simulink model "EPT"  (R2019b)
settings: Solver=FixedStepDiscrete  StartTime=0.0  StopTime=5  FixedStep=0.005  RelTol=1e-3  EnableMultiTasking=on
PreLoadFcn:
  | try, model_open; catch, disp('Error occurred while executing model pre-load callback: model_open.m'); disp('Please assure that the MATLAB working directory is set to the model directory before opening.'); end
InitFcn:
  | try, model_open; catch, end
undefined symbols (not defined in the file or in its folder): Bridge, GCM, H, ln, raptor_get_param_eval, raptor_get_safe_string, raptor_xcp_function
libraries: Raptor_lib x2810, simulink x374, hdlsllib x19
(part 13 of 45)

== system EPT/Foreground_TimeBase_5ms/CAN/CAN1_exec/BCU vs RMDA-BMS/Remote DAG2-5E6 ==
  Trigger : TriggerPort  VariantControl=Variant  PortDimensions=1
  Bitwise Operator : simulink/Logic and Bit Operations/Bitwise Operator  logicop=AND  UseBitMask=on  BitMask=hex2dec('f0')  BitMaskRealWorld=Stored Integer
  Bitwise Operator1 : simulink/Logic and Bit Operations/Bitwise Operator  logicop=AND  UseBitMask=on  BitMask=hex2dec('0f')  BitMaskRealWorld=Stored Integer
  Data Type Conversion{,1..5} (6 alike) : DataTypeConversion
  Fcn1 : Fcn  Expr=(u(1)+12.5)/0.5
  Shift Arithmetic1 : ArithShift  BitShiftNumber=4  BitShiftDirection=Right
  raptor_can_txmsg : Raptor_lib/CAN/raptor_can_txmsg  canDefinition=struct('dbcFile', 'BCUvsRMDA_CMU.dbc','message', 'RemoteDAG_5E6','comment', '','signals', {{'CMU2_EW_Level3_Hbyte','CMU2_EW_Level3_Lbyte','CMU2_FCC','CMU2_Mode','CMU2_RSOC','CMU2_Rcap'}},'enabled', [ 1 1 1 1 1 1;],'canBus', '''CAN1''','messageID', [ 1510;],'idMask', [ 536870911;],'payloadMask', [],'payloadValue', [],'period', [ 0;],'mailbox', '','queueSize', [ 1;],'label', [ 0;],'ver', [ 2;],'showID', [ 0;],'showRaw', [ 0;],'fill', [ 0;],'editID', [ 0;],'signalOrder', [ 1;])  canBus='CAN1'  queueSize=1  payloadMask=[]  payloadValue=[]  period=0  showID=0  label=0  idMask=hex2dec('1FFFFFFF')  fill=0  id=1510  showRaw=0  signalOrder=1  signalInfo={{struct('Name', 'CMU2_Mode','Startbit', [ 0;],'SignalSize', [ 8;],'ByteOrder', 'BigEndian','ValueType', 'UNSIGNED','Class', 'uint8','Signed', [ 0;],'Factor', [ 1;],'Offset', [ 0;],'Min', [ 0;],'Max', [ 0;],'Units', '','Comment', '','StartBit', [ 0;]),struct('Name', 'CMU2_EW_Level3_Hbyte','Startbit', [ 0;],'SignalSize', [ 8;],'ByteOrder', 'BigEndian','ValueType', 'UNSIGNED','Class', 'uint8','Signed', [ 0;],'Factor', [ 1;],'Offset', [ 0;],'Min', [ 0;],'Max', [ 0;],'Units', '','Comment', '','StartBit', [ 8;]),struct('Name', 'CMU2_EW_Level3_Lbyte','Startbit', [ 0;],'SignalSize', [ 8;],'ByteOrder', 'BigEndian','ValueType', 'UNSIGNED','Class', 'uint8','Signed', [ 0;],'Factor', [ 1;],'Offset', [ 0;],'Min', [ 0;],'Max', [ 0;],'Units', '','Comment', '','StartBit', [ 16;]),struct('Name', 'CMU2_FCC','Startbit', [ 0;],'SignalSize', [ 8;],'ByteOrder', 'BigEndian','ValueType', 'UNSIGNED','Class', 'uint8','Signed', [ 0;],'Factor', [ 1;],'Offset', [ 0;],'Min', [ 0;],'Max', [ 0;],'Units', '','Comment', '','StartBit', [ 32;]),struct('Name', 'CMU2_Rcap','Startbit', [ 0;],'SignalSize', [ 8;],'ByteOrder', 'BigEndian','ValueType', 'UNSIGNED','Class', 'uint8','Signed', [ 0;],'Factor', [ 1;],'Offset', [ 0;],'Min', [ 0;],'Max', [ 0;],'Units', '','Comment', '','StartBit', [ 40;]),struct('Name', 'CMU2_RSOC','Startbit', [ 0;],'SignalSize', [ 8;],'ByteOrder', 'BigEndian','ValueType', 'UNSIGNED','Class', 'uint8','Signed', [ 0;],'Factor', [ 1;],'Offset', [ 0;],'Min', [ 0;],'Max', [ 0;],'Units', '','Comment', '','StartBit', [ 48;])}}
      settings: SourceProductName=Raptor
  raptor_data_read2 : Raptor_lib/Data Storage/raptor_data_read  dataName='Rx_0x200B2A2_FCC'  dataShape=Scalar  idxSource=Input  idxRow=1  idxCol=1
      settings: SourceProductName=Raptor
  raptor_data_read3 : Raptor_lib/Data Storage/raptor_data_read  dataName='Rx_0x200B0A2_CMU2_Status'  dataShape=Scalar  idxSource=Input  idxRow=1  idxCol=1
      settings: SourceProductName=Raptor
  raptor_data_read4 : Raptor_lib/Data Storage/raptor_data_read  dataName='Rx_0x200B2A2_RC'  dataShape=Scalar  idxSource=Input  idxRow=1  idxCol=1
      settings: SourceProductName=Raptor
  raptor_data_read5 : Raptor_lib/Data Storage/raptor_data_read  dataName='Rx_0x200B2A2_RSOC'  dataShape=Scalar  idxSource=Input  idxRow=1  idxCol=1
      settings: SourceProductName=Raptor
  raptor_data_read6 : Raptor_lib/Data Storage/raptor_data_read  dataName='Rx_0x200BAA2_Event3_Error_Code'  dataShape=Scalar  idxSource=Input  idxRow=1  idxCol=1
      settings: SourceProductName=Raptor
  wires:
  Data Type Conversion/1 -> Data Type Conversion2/1
  Shift Arithmetic1/1 -> Data Type Conversion1/1
  raptor_data_read6/1 -> Bitwise Operator/1, Bitwise Operator1/1
  Bitwise Operator1/1 -> Data Type Conversion/1
  raptor_data_read3/1 -> raptor_can_txmsg/4
  Bitwise Operator/1 -> Shift Arithmetic1/1
  raptor_data_read2/1 -> Data Type Conversion5/1
  Data Type Conversion2/1 -> raptor_can_txmsg/2
  Data Type Conversion1/1 -> raptor_can_txmsg/1
  raptor_data_read5/1 -> Fcn1/1
  Data Type Conversion3/1 -> raptor_can_txmsg/6
  raptor_data_read4/1 -> Data Type Conversion3/1
  Data Type Conversion4/1 -> raptor_can_txmsg/5
  Data Type Conversion5/1 -> raptor_can_txmsg/3
  Fcn1/1 -> Data Type Conversion4/1

== system EPT/Foreground_TimeBase_5ms/CAN/CAN1_exec/BCU vs RMDA-BMS/Remote DAG2-5E7 ==
  Trigger : TriggerPort  VariantControl=Variant  PortDimensions=1
  Data Type Conversion{1..4} (4 alike) : DataTypeConversion
  Fcn1 : Fcn  Expr=(u(1)-2)/0.01
  Fcn2 : Fcn  Expr=(u(1)-2)/0.01
  Fcn3 : Fcn  Expr=(u(1)+40)/0.5
  Fcn4 : Fcn  Expr=(u(1)+40)/0.5
  raptor_can_txmsg : Raptor_lib/CAN/raptor_can_txmsg  canDefinition=struct('dbcFile', 'BCUvsRMDA_CMU.dbc','message', 'RemoteDAG_5E7','comment', '','signals', {{'CMU2_Ibp','CMU2_Tcell_Max','CMU2_Tcell_Min','CMU2_Vbp','CMU2_Vcell_Max','CMU2_Vcell_Min'}},'enabled', [ 1 1 1 1 1 1;],'canBus', '''CAN1''','messageID', [ 1511;],'idMask', [ 536870911;],'payloadMask', [],'payloadValue', [],'period', [ 0;],'mailbox', '','queueSize', [ 1;],'label', [ 0;],'ver', [ 2;],'showID', [ 0;],'showRaw', [ 0;],'fill', [ 0;],'editID', [ 0;],'signalOrder', [ 1;])  canBus='CAN1'  queueSize=1  payloadMask=[]  payloadValue=[]  period=0  showID=0  label=0  idMask=hex2dec('1FFFFFFF')  fill=0  id=1511  showRaw=0  signalOrder=1  signalInfo={{struct('Name', 'CMU2_Ibp','Startbit', [ 0;],'SignalSize', [ 16;],'ByteOrder', 'BigEndian','ValueType', 'UNSIGNED','Class', 'uint16','Signed', [ 0;],'Factor', [ 0.02;],'Offset', [ -500;],'Min', [ 0;],'Max', [ 0;],'Units', '','Comment', '','StartBit', [ 8;]),struct('Name', 'CMU2_Vbp','Startbit', [ 0;],'SignalSize', [ 16;],'ByteOrder', 'BigEndian','ValueType', 'UNSIGNED','Class', 'uint16','Signed', [ 0;],'Factor', [ 0.01;],'Offset', [ 0;],'Min', [ 0;],'Max', [ 0;],'Units', '','Comment', '','StartBit', [ 24;]),struct('Name', 'CMU2_Vcell_Max','Startbit', [ 0;],'SignalSize', [ 8;],'ByteOrder', 'BigEndian','ValueType', 'UNSIGNED','Class', 'uint8','Signed', [ 0;],'Factor', [ 1;],'Offset', [ 0;],'Min', [ 0;],'Max', [ 0;],'Units', '','Comment', '','StartBit', [ 32;]),struct('Name', 'CMU2_Vcell_Min','Startbit', [ 0;],'SignalSize', [ 8;],'ByteOrder', 'BigEndian','ValueType', 'UNSIGNED','Class', 'uint8','Signed', [ 0;],'Factor', [ 1;],'Offset', [ 0;],'Min', [ 0;],'Max', [ 0;],'Units', '','Comment', '','StartBit', [ 40;]),struct('Name', 'CMU2_Tcell_Max','Startbit', [ 0;],'SignalSize', [ 8;],'ByteOrder', 'BigEndian','ValueType', 'UNSIGNED','Class', 'uint8','Signed', [ 0;],'Factor', [ 1;],'Offset', [ 0;],'Min', [ 0;],'Max', [ 0;],'Units', '','Comment', '','StartBit', [ 48;]),struct('Name', 'CMU2_Tcell_Min','Startbit', [ 0;],'SignalSize', [ 8;],'ByteOrder', 'BigEndian','ValueType', 'UNSIGNED','Class', 'uint8','Signed', [ 0;],'Factor', [ 1;],'Offset', [ 0;],'Min', [ 0;],'Max', [ 0;],'Units', '','Comment', '','StartBit', [ 56;])}}
      settings: SourceProductName=Raptor
  raptor_data_read : Raptor_lib/Data Storage/raptor_data_read  dataName='Rx_0x200B0A2_Max_Cell_Volt'  dataShape=Scalar  idxSource=Input  idxRow=1  idxCol=1
      settings: SourceProductName=Raptor
  raptor_data_read1 : Raptor_lib/Data Storage/raptor_data_read  dataName='Rx_0x200B0A2_Min_Cell_Volt'  dataShape=Scalar  idxSource=Input  idxRow=1  idxCol=1
      settings: SourceProductName=Raptor
  raptor_data_read2 : Raptor_lib/Data Storage/raptor_data_read  dataName='Rx_0x200B1A2_Min_Cell_Temp'  dataShape=Scalar  idxSource=Input  idxRow=1  idxCol=1
      settings: SourceProductName=Raptor
  raptor_data_read3 : Raptor_lib/Data Storage/raptor_data_read  dataName='Rx_0x200B0A2_Battery_Current'  dataShape=Scalar  idxSource=Input  idxRow=1  idxCol=1
      settings: SourceProductName=Raptor
  raptor_data_read4 : Raptor_lib/Data Storage/raptor_data_read  dataName='Rx_0x200B1A2_BatteryVolt'  dataShape=Scalar  idxSource=Input  idxRow=1  idxCol=1
      settings: SourceProductName=Raptor
  raptor_data_read5 : Raptor_lib/Data Storage/raptor_data_read  dataName='Rx_0x200B1A2_Max_Cell_Temp'  dataShape=Scalar  idxSource=Input  idxRow=1  idxCol=1
      settings: SourceProductName=Raptor
  wires:
  raptor_data_read4/1 -> raptor_can_txmsg/4
  raptor_data_read3/1 -> raptor_can_txmsg/1
  Fcn1/1 -> Data Type Conversion4/1
  raptor_data_read1/1 -> Fcn1/1
  Fcn2/1 -> Data Type Conversion1/1
  raptor_data_read/1 -> Fcn2/1
  Data Type Conversion1/1 -> raptor_can_txmsg/5
  Data Type Conversion4/1 -> raptor_can_txmsg/6
  Fcn3/1 -> Data Type Conversion2/1
  Data Type Conversion2/1 -> raptor_can_txmsg/2
  raptor_data_read5/1 -> Fcn3/1
  Fcn4/1 -> Data Type Conversion3/1
  Data Type Conversion3/1 -> raptor_can_txmsg/3
  raptor_data_read2/1 -> Fcn4/1

== system EPT/Foreground_TimeBase_5ms/CAN/CAN1_exec/BCU vs RMDA-BMS/Remote DAG2-5E8 ==
  Trigger : TriggerPort  VariantControl=Variant  PortDimensions=1
  Data Type Conversion{1..8} (8 alike) : DataTypeConversion
  Fcn{,1..7} (8 alike) : Fcn  Expr=(u(1)-2)/0.01
  raptor_can_txmsg : Raptor_lib/CAN/raptor_can_txmsg  canDefinition=struct('dbcFile', 'BCUvsRMDA_CMU.dbc','message', 'RemoteDAG_5E8','comment', '','signals', {{'CMU2_Vcell_V01','CMU2_Vcell_V02','CMU2_Vcell_V03','CMU2_Vcell_V04','CMU2_Vcell_V05','CMU2_Vcell_V06','CMU2_Vcell_V07','CMU2_Vcell_V08'}},'enabled', [ 1 1 1 1 1 1 1 1;],'canBus', '''CAN1''','messageID', [ 1512;],'idMask', [ 536870911;],'payloadMask', [],'payloadValue', [],'period', [ 0;],'mailbox', '','queueSize', [ 1;],'label', [ 0;],'ver', [ 2;],'showID', [ 0;],'showRaw', [ 0;],'fill', [ 0;],'editID', [ 0;],'signalOrder', [ 1;])  canBus='CAN1'  queueSize=1  payloadMask=[]  payloadValue=[]  period=0  showID=0  label=0  idMask=hex2dec('1FFFFFFF')  fill=0  id=1512  showRaw=0  signalOrder=1  signalInfo={{struct('Name', 'CMU2_Vcell_V01','Startbit', [ 0;],'SignalSize', [ 8;],'ByteOrder', 'BigEndian','ValueType', 'UNSIGNED','Class', 'uint8','Signed', [ 0;],'Factor', [ 1;],'Offset', [ 0;],'Min', [ 0;],'Max', [ 0;],'Units', '','Comment', '','StartBit', [ 0;]),struct('Name', 'CMU2_Vcell_V02','Startbit', [ 0;],'SignalSize', [ 8;],'ByteOrder', 'BigEndian','ValueType', 'UNSIGNED','Class', 'uint8','Signed', [ 0;],'Factor', [ 1;],'Offset', [ 0;],'Min', [ 0;],'Max', [ 0;],'Units', '','Comment', '','StartBit', [ 8;]),struct('Name', 'CMU2_Vcell_V03','Startbit', [ 0;],'SignalSize', [ 8;],'ByteOrder', 'BigEndian','ValueType', 'UNSIGNED','Class', 'uint8','Signed', [ 0;],'Factor', [ 1;],'Offset', [ 0;],'Min', [ 0;],'Max', [ 0;],'Units', '','Comment', '','StartBit', [ 16;]),struct('Name', 'CMU2_Vcell_V04','Startbit', [ 0;],'SignalSize', [ 8;],'ByteOrder', 'BigEndian','ValueType', 'UNSIGNED','Class', 'uint8','Signed', [ 0;],'Factor', [ 1;],'Offset', [ 0;],'Min', [ 0;],'Max', [ 0;],'Units', '','Comment', '','StartBit', [ 24;]),struct('Name', 'CMU2_Vcell_V05','Startbit', [ 0;],'SignalSize', [ 8;],'ByteOrder', 'BigEndian','ValueType', 'UNSIGNED','Class', 'uint8','Signed', [ 0;],'Factor', [ 1;],'Offset', [ 0;],'Min', [ 0;],'Max', [ 0;],'Units', '','Comment', '','StartBit', [ 32;]),struct('Name', 'CMU2_Vcell_V06','Startbit', [ 0;],'SignalSize', [ 8;],'ByteOrder', 'BigEndian','ValueType', 'UNSIGNED','Class', 'uint8','Signed', [ 0;],'Factor', [ 1;],'Offset', [ 0;],'Min', [ 0;],'Max', [ 0;],'Units', '','Comment', '','StartBit', [ 40;]),struct('Name', 'CMU2_Vcell_V07','Startbit', [ 0;],'SignalSize', [ 8;],'ByteOrder', 'BigEndian','ValueType', 'UNSIGNED','Class', 'uint8','Signed', [ 0;],'Factor', [ 1;],'Offset', [ 0;],'Min', [ 0;],'Max', [ 0;],'Units', '','Comment', '','StartBit', [ 48;]),struct('Name', 'CMU2_Vcell_V08','Startbit', [ 0;],'SignalSize', [ 8;],'ByteOrder', 'BigEndian','ValueType', 'UNSIGNED','Class', 'uint8','Signed', [ 0;],'Factor', [ 1;],'Offset', [ 0;],'Min', [ 0;],'Max', [ 0;],'Units', '','Comment', '','StartBit', [ 56;])}}
      settings: SourceProductName=Raptor
  raptor_data_read : Raptor_lib/Data Storage/raptor_data_read  dataName='Rx_0x200C0A2_Cell_1_Volt'  dataShape=Scalar  idxSource=Input  idxRow=1  idxCol=1
      settings: SourceProductName=Raptor
  raptor_data_read1 : Raptor_lib/Data Storage/raptor_data_read  dataName='Rx_0x200C0A2_Cell_2_Volt'  dataShape=Scalar  idxSource=Input  idxRow=1  idxCol=1
      settings: SourceProductName=Raptor
  raptor_data_read2 : Raptor_lib/Data Storage/raptor_data_read  dataName='Rx_0x200C0A2_Cell_3_Volt'  dataShape=Scalar  idxSource=Input  idxRow=1  idxCol=1
      settings: SourceProductName=Raptor
  raptor_data_read3 : Raptor_lib/Data Storage/raptor_data_read  dataName='Rx_0x200C0A2_Cell_4_Volt'  dataShape=Scalar  idxSource=Input  idxRow=1  idxCol=1
      settings: SourceProductName=Raptor
  raptor_data_read4 : Raptor_lib/Data Storage/raptor_data_read  dataName='Rx_0x200C1A2_Cell_5_Volt'  dataShape=Scalar  idxSource=Input  idxRow=1  idxCol=1
      settings: SourceProductName=Raptor
  raptor_data_read5 : Raptor_lib/Data Storage/raptor_data_read  dataName='Rx_0x200C1A2_Cell_6_Volt'  dataShape=Scalar  idxSource=Input  idxRow=1  idxCol=1
      settings: SourceProductName=Raptor
  raptor_data_read6 : Raptor_lib/Data Storage/raptor_data_read  dataName='Rx_0x200C1A2_Cell_7_Volt'  dataShape=Scalar  idxSource=Input  idxRow=1  idxCol=1
      settings: SourceProductName=Raptor
  raptor_data_read7 : Raptor_lib/Data Storage/raptor_data_read  dataName='Rx_0x200C1A2_Cell_8_Volt'  dataShape=Scalar  idxSource=Input  idxRow=1  idxCol=1
      settings: SourceProductName=Raptor
  wires:
  raptor_data_read6/1 -> Fcn6/1
  raptor_data_read2/1 -> Fcn2/1
  raptor_data_read5/1 -> Fcn5/1
  raptor_data_read1/1 -> Fcn1/1
  raptor_data_read/1 -> Fcn/1
  Data Type Conversion6/1 -> raptor_can_txmsg/4
  Data Type Conversion7/1 -> raptor_can_txmsg/3
  Data Type Conversion8/1 -> raptor_can_txmsg/2
  Data Type Conversion4/1 -> raptor_can_txmsg/1
  Data Type Conversion2/1 -> raptor_can_txmsg/7
  Data Type Conversion1/1 -> raptor_can_txmsg/6
  raptor_data_read3/1 -> Fcn3/1
  Fcn1/1 -> Data Type Conversion8/1
  Fcn7/1 -> Data Type Conversion3/1
  raptor_data_read4/1 -> Fcn4/1
  Fcn2/1 -> Data Type Conversion7/1
  Fcn6/1 -> Data Type Conversion2/1
  Fcn4/1 -> Data Type Conversion5/1
  Fcn5/1 -> Data Type Conversion1/1
  Data Type Conversion5/1 -> raptor_can_txmsg/5
  Data Type Conversion3/1 -> raptor_can_txmsg/8
  Fcn3/1 -> Data Type Conversion6/1
  Fcn/1 -> Data Type Conversion4/1
  raptor_data_read7/1 -> Fcn7/1

== system EPT/Foreground_TimeBase_5ms/CAN/CAN1_exec/BCU vs RMDA-BMS/Remote DAG2-5E9 ==
  Trigger : TriggerPort  VariantControl=Variant  PortDimensions=1
  Data Type Conversion{1..8} (8 alike) : DataTypeConversion
  Fcn{,1..7} (8 alike) : Fcn  Expr=(u(1)-2)/0.01
  raptor_can_txmsg : Raptor_lib/CAN/raptor_can_txmsg  canDefinition=struct('dbcFile', 'BCUvsRMDA_CMU.dbc','message', 'RemoteDAG_5E9','comment', '','signals', {{'CMU2_Vcell_V09','CMU2_Vcell_V10','CMU2_Vcell_V11','CMU2_Vcell_V12','CMU2_Vcell_V13','CMU2_Vcell_V14','CMU2_Vcell_V15','CMU2_Vcell_V16'}},'enabled', [ 1 1 1 1 1 1 1 1;],'canBus', '''CAN1''','messageID', [ 1513;],'idMask', [ 536870911;],'payloadMask', [],'payloadValue', [],'period', [ 0;],'mailbox', '','queueSize', [ 1;],'label', [ 0;],'ver', [ 2;],'showID', [ 0;],'showRaw', [ 0;],'fill', [ 0;],'editID', [ 0;],'signalOrder', [ 1;])  canBus='CAN1'  queueSize=1  payloadMask=[]  payloadValue=[]  period=0  showID=0  label=0  idMask=hex2dec('1FFFFFFF')  fill=0  id=1513  showRaw=0  signalOrder=1  signalInfo={{struct('Name', 'CMU2_Vcell_V09','Startbit', [ 0;],'SignalSize', [ 8;],'ByteOrder', 'BigEndian','ValueType', 'UNSIGNED','Class', 'uint8','Signed', [ 0;],'Factor', [ 1;],'Offset', [ 0;],'Min', [ 0;],'Max', [ 0;],'Units', '','Comment', '','StartBit', [ 0;]),struct('Name', 'CMU2_Vcell_V10','Startbit', [ 0;],'SignalSize', [ 8;],'ByteOrder', 'BigEndian','ValueType', 'UNSIGNED','Class', 'uint8','Signed', [ 0;],'Factor', [ 1;],'Offset', [ 0;],'Min', [ 0;],'Max', [ 0;],'Units', '','Comment', '','StartBit', [ 8;]),struct('Name', 'CMU2_Vcell_V11','Startbit', [ 0;],'SignalSize', [ 8;],'ByteOrder', 'BigEndian','ValueType', 'UNSIGNED','Class', 'uint8','Signed', [ 0;],'Factor', [ 1;],'Offset', [ 0;],'Min', [ 0;],'Max', [ 0;],'Units', '','Comment', '','StartBit', [ 16;]),struct('Name', 'CMU2_Vcell_V12','Startbit', [ 0;],'SignalSize', [ 8;],'ByteOrder', 'BigEndian','ValueType', 'UNSIGNED','Class', 'uint8','Signed', [ 0;],'Factor', [ 1;],'Offset', [ 0;],'Min', [ 0;],'Max', [ 0;],'Units', '','Comment', '','StartBit', [ 24;]),struct('Name', 'CMU2_Vcell_V13','Startbit', [ 0;],'SignalSize', [ 8;],'ByteOrder', 'BigEndian','ValueType', 'UNSIGNED','Class', 'uint8','Signed', [ 0;],'Factor', [ 1;],'Offset', [ 0;],'Min', [ 0;],'Max', [ 0;],'Units', '','Comment', '','StartBit', [ 32;]),struct('Name', 'CMU2_Vcell_V14','Startbit', [ 0;],'SignalSize', [ 8;],'ByteOrder', 'BigEndian','ValueType', 'UNSIGNED','Class', 'uint8','Signed', [ 0;],'Factor', [ 1;],'Offset', [ 0;],'Min', [ 0;],'Max', [ 0;],'Units', '','Comment', '','StartBit', [ 40;]),struct('Name', 'CMU2_Vcell_V15','Startbit', [ 0;],'SignalSize', [ 8;],'ByteOrder', 'BigEndian','ValueType', 'UNSIGNED','Class', 'uint8','Signed', [ 0;],'Factor', [ 1;],'Offset', [ 0;],'Min', [ 0;],'Max', [ 0;],'Units', '','Comment', '','StartBit', [ 48;]),struct('Name', 'CMU2_Vcell_V16','Startbit', [ 0;],'SignalSize', [ 8;],'ByteOrder', 'BigEndian','ValueType', 'UNSIGNED','Class', 'uint8','Signed', [ 0;],'Factor', [ 1;],'Offset', [ 0;],'Min', [ 0;],'Max', [ 0;],'Units', '','Comment', '','StartBit', [ 56;])}}
      settings: SourceProductName=Raptor
  raptor_data_read : Raptor_lib/Data Storage/raptor_data_read  dataName='Rx_0x200C2A1_Cell_10_Volt'  dataShape=Scalar  idxSource=Input  idxRow=1  idxCol=1
      settings: SourceProductName=Raptor
  raptor_data_read1 : Raptor_lib/Data Storage/raptor_data_read  dataName='Rx_0x200C2A1_Cell_11_Volt'  dataShape=Scalar  idxSource=Input  idxRow=1  idxCol=1
      settings: SourceProductName=Raptor
  raptor_data_read2 : Raptor_lib/Data Storage/raptor_data_read  dataName='Rx_0x200C2A1_Cell_12_Volt'  dataShape=Scalar  idxSource=Input  idxRow=1  idxCol=1
      settings: SourceProductName=Raptor
  raptor_data_read3 : Raptor_lib/Data Storage/raptor_data_read  dataName='Rx_0x200C3A1_Cell_13_Volt'  dataShape=Scalar  idxSource=Input  idxRow=1  idxCol=1
      settings: SourceProductName=Raptor
  raptor_data_read4 : Raptor_lib/Data Storage/raptor_data_read  dataName='Rx_0x200C2A1_Cell_9_Volt'  dataShape=Scalar  idxSource=Input  idxRow=1  idxCol=1
      settings: SourceProductName=Raptor
  raptor_data_read5 : Raptor_lib/Data Storage/raptor_data_read  dataName='Rx_0x200C3A1_Cell_14_Volt'  dataShape=Scalar  idxSource=Input  idxRow=1  idxCol=1
      settings: SourceProductName=Raptor
  raptor_data_read6 : Raptor_lib/Data Storage/raptor_data_read  dataName='Rx_0x200C3A1_Cell_15_Volt'  dataShape=Scalar  idxSource=Input  idxRow=1  idxCol=1
      settings: SourceProductName=Raptor
  raptor_data_read7 : Raptor_lib/Data Storage/raptor_data_read  dataName='Rx_0x200C3A1_Cell_16_Volt'  dataShape=Scalar  idxSource=Input  idxRow=1  idxCol=1
      settings: SourceProductName=Raptor
  wires:
  raptor_data_read7/1 -> Fcn7/1
  raptor_data_read4/1 -> Fcn/1
  Fcn5/1 -> Data Type Conversion1/1
  Fcn6/1 -> Data Type Conversion2/1
  Fcn3/1 -> Data Type Conversion6/1
  raptor_data_read5/1 -> Fcn5/1
  raptor_data_read1/1 -> Fcn2/1
  raptor_data_read6/1 -> Fcn6/1
  Fcn4/1 -> Data Type Conversion5/1
  Fcn/1 -> Data Type Conversion4/1
  raptor_data_read2/1 -> Fcn3/1
  Fcn1/1 -> Data Type Conversion8/1
  Fcn2/1 -> Data Type Conversion7/1
  raptor_data_read3/1 -> Fcn4/1
  Fcn7/1 -> Data Type Conversion3/1
  raptor_data_read/1 -> Fcn1/1
  Data Type Conversion2/1 -> raptor_can_txmsg/7
  Data Type Conversion1/1 -> raptor_can_txmsg/6
  Data Type Conversion5/1 -> raptor_can_txmsg/5
  Data Type Conversion6/1 -> raptor_can_txmsg/4
  Data Type Conversion7/1 -> raptor_can_txmsg/3
  Data Type Conversion8/1 -> raptor_can_txmsg/2
  Data Type Conversion4/1 -> raptor_can_txmsg/1

== system EPT/Foreground_TimeBase_5ms/CAN/CAN1_exec/BCU vs RMDA-BMS/Remote DAG2-5EA ==
  Trigger : TriggerPort  VariantControl=Variant  PortDimensions=1
  Data Type Conversion{1..8} (8 alike) : DataTypeConversion
  Fcn{1..8} (8 alike) : Fcn  Expr=(u(1)+40)/0.5
  raptor_can_txmsg : Raptor_lib/CAN/raptor_can_txmsg  canDefinition=struct('dbcFile', 'BCUvsRMDA_CMU.dbc','message', 'RemoteDAG_5EA','comment', '','signals', {{'CMU2_Tcell_T01','CMU2_Tcell_T02','CMU2_Tcell_T03','CMU2_Tcell_T04','CMU2_Tcell_T05','CMU2_Tcell_T06','CMU2_Tcell_T07','CMU2_Tcell_T08'}},'enabled', [ 1 1 1 1 1 1 1 1;],'canBus', '''CAN1''','messageID', [ 1514;],'idMask', [ 536870911;],'payloadMask', [],'payloadValue', [],'period', [ 0;],'mailbox', '','queueSize', [ 1;],'label', [ 0;],'ver', [ 2;],'showID', [ 0;],'showRaw', [ 0;],'fill', [ 0;],'editID', [ 0;],'signalOrder', [ 1;])  canBus='CAN1'  queueSize=1  payloadMask=[]  payloadValue=[]  period=0  showID=0  label=0  idMask=hex2dec('1FFFFFFF')  fill=0  id=1514  showRaw=0  signalOrder=1  signalInfo={{struct('Name', 'CMU2_Tcell_T01','Startbit', [ 0;],'SignalSize', [ 8;],'ByteOrder', 'BigEndian','ValueType', 'UNSIGNED','Class', 'uint8','Signed', [ 0;],'Factor', [ 1;],'Offset', [ 0;],'Min', [ 0;],'Max', [ 0;],'Units', '','Comment', '','StartBit', [ 0;]),struct('Name', 'CMU2_Tcell_T02','Startbit', [ 0;],'SignalSize', [ 8;],'ByteOrder', 'BigEndian','ValueType', 'UNSIGNED','Class', 'uint8','Signed', [ 0;],'Factor', [ 1;],'Offset', [ 0;],'Min', [ 0;],'Max', [ 0;],'Units', '','Comment', '','StartBit', [ 8;]),struct('Name', 'CMU2_Tcell_T03','Startbit', [ 0;],'SignalSize', [ 8;],'ByteOrder', 'BigEndian','ValueType', 'UNSIGNED','Class', 'uint8','Signed', [ 0;],'Factor', [ 1;],'Offset', [ 0;],'Min', [ 0;],'Max', [ 0;],'Units', '','Comment', '','StartBit', [ 16;]),struct('Name', 'CMU2_Tcell_T04','Startbit', [ 0;],'SignalSize', [ 8;],'ByteOrder', 'BigEndian','ValueType', 'UNSIGNED','Class', 'uint8','Signed', [ 0;],'Factor', [ 1;],'Offset', [ 0;],'Min', [ 0;],'Max', [ 0;],'Units', '','Comment', '','StartBit', [ 24;]),struct('Name', 'CMU2_Tcell_T05','Startbit', [ 0;],'SignalSize', [ 8;],'ByteOrder', 'BigEndian','ValueType', 'UNSIGNED','Class', 'uint8','Signed', [ 0;],'Factor', [ 1;],'Offset', [ 0;],'Min', [ 0;],'Max', [ 0;],'Units', '','Comment', '','StartBit', [ 32;]),struct('Name', 'CMU2_Tcell_T06','Startbit', [ 0;],'SignalSize', [ 8;],'ByteOrder', 'BigEndian','ValueType', 'UNSIGNED','Class', 'uint8','Signed', [ 0;],'Factor', [ 1;],'Offset', [ 0;],'Min', [ 0;],'Max', [ 0;],'Units', '','Comment', '','StartBit', [ 40;]),struct('Name', 'CMU2_Tcell_T07','Startbit', [ 0;],'SignalSize', [ 8;],'ByteOrder', 'BigEndian','ValueType', 'UNSIGNED','Class', 'uint8','Signed', [ 0;],'Factor', [ 1;],'Offset', [ 0;],'Min', [ 0;],'Max', [ 0;],'Units', '','Comment', '','StartBit', [ 48;]),struct('Name', 'CMU2_Tcell_T08','Startbit', [ 0;],'SignalSize', [ 8;],'ByteOrder', 'BigEndian','ValueType', 'UNSIGNED','Class', 'uint8','Signed', [ 0;],'Factor', [ 1;],'Offset', [ 0;],'Min', [ 0;],'Max', [ 0;],'Units', '','Comment', '','StartBit', [ 56;])}}
      settings: SourceProductName=Raptor
  raptor_data_read : Raptor_lib/Data Storage/raptor_data_read  dataName='Rx_0x200C4A2_Cell_1_Temp'  dataShape=Scalar  idxSource=Input  idxRow=1  idxCol=1
      settings: SourceProductName=Raptor
  raptor_data_read1 : Raptor_lib/Data Storage/raptor_data_read  dataName='Rx_0x200C4A2_Cell_2_Temp'  dataShape=Scalar  idxSource=Input  idxRow=1  idxCol=1
      settings: SourceProductName=Raptor
  raptor_data_read2 : Raptor_lib/Data Storage/raptor_data_read  dataName='Rx_0x200C4A2_Cell_3_Temp'  dataShape=Scalar  idxSource=Input  idxRow=1  idxCol=1
      settings: SourceProductName=Raptor
  raptor_data_read3 : Raptor_lib/Data Storage/raptor_data_read  dataName='Rx_0x200C4A2_Cell_4_Temp'  dataShape=Scalar  idxSource=Input  idxRow=1  idxCol=1
      settings: SourceProductName=Raptor
  raptor_data_read4 : Raptor_lib/Data Storage/raptor_data_read  dataName='Rx_0x200C5A2_Cell_5_Temp'  dataShape=Scalar  idxSource=Input  idxRow=1  idxCol=1
      settings: SourceProductName=Raptor
  raptor_data_read5 : Raptor_lib/Data Storage/raptor_data_read  dataName='Rx_0x200C5A2_Cell_6_Temp'  dataShape=Scalar  idxSource=Input  idxRow=1  idxCol=1
      settings: SourceProductName=Raptor
  raptor_data_read6 : Raptor_lib/Data Storage/raptor_data_read  dataName='Rx_0x200C5A2_Cell_7_Temp'  dataShape=Scalar  idxSource=Input  idxRow=1  idxCol=1
      settings: SourceProductName=Raptor
  raptor_data_read7 : Raptor_lib/Data Storage/raptor_data_read  dataName='Rx_0x200C5A2_Cell_8_Temp'  dataShape=Scalar  idxSource=Input  idxRow=1  idxCol=1
      settings: SourceProductName=Raptor
  wires:
  raptor_data_read7/1 -> Fcn8/1
  Data Type Conversion5/1 -> raptor_can_txmsg/5
  Fcn4/1 -> Data Type Conversion4/1
  Fcn1/1 -> Data Type Conversion1/1
  Fcn8/1 -> Data Type Conversion8/1
  Data Type Conversion1/1 -> raptor_can_txmsg/2
  Data Type Conversion4/1 -> raptor_can_txmsg/4
  Data Type Conversion7/1 -> raptor_can_txmsg/7
  Fcn3/1 -> Data Type Conversion2/1
  Fcn6/1 -> Data Type Conversion6/1
  Fcn7/1 -> Data Type Conversion7/1
  raptor_data_read1/1 -> Fcn1/1
  Data Type Conversion6/1 -> raptor_can_txmsg/6
  raptor_data_read6/1 -> Fcn7/1
  Fcn2/1 -> Data Type Conversion3/1
  Data Type Conversion2/1 -> raptor_can_txmsg/3
  Data Type Conversion3/1 -> raptor_can_txmsg/1
  Fcn5/1 -> Data Type Conversion5/1
  Data Type Conversion8/1 -> raptor_can_txmsg/8
  raptor_data_read4/1 -> Fcn5/1
  raptor_data_read2/1 -> Fcn3/1
  raptor_data_read5/1 -> Fcn6/1
  raptor_data_read/1 -> Fcn2/1
  raptor_data_read3/1 -> Fcn4/1

== system EPT/Foreground_TimeBase_5ms/CAN/CAN1_exec/BCU vs RMDA-BMS/Remote DAG2-5EB ==
  Trigger : TriggerPort  VariantControl=Variant  PortDimensions=1
  Data Type Conversion{1..8} (8 alike) : DataTypeConversion
  Fcn{1..8} (8 alike) : Fcn  Expr=(u(1)+40)/0.5
  raptor_can_txmsg : Raptor_lib/CAN/raptor_can_txmsg  canDefinition=struct('dbcFile', 'BCUvsRMDA_CMU.dbc','message', 'RemoteDAG_5EB','comment', '','signals', {{'CMU2_Tcell_T09','CMU2_Tcell_T10','CMU2_Tcell_T11','CMU2_Tcell_T12','CMU2_Tcell_T13','CMU2_Tcell_T14','CMU2_Tcell_T15','CMU2_Tcell_T16'}},'enabled', [ 1 1 1 1 1 1 1 1;],'canBus', '''CAN1''','messageID', [ 1515;],'idMask', [ 536870911;],'payloadMask', [],'payloadValue', [],'period', [ 0;],'mailbox', '','queueSize', [ 1;],'label', [ 0;],'ver', [ 2;],'showID', [ 0;],'showRaw', [ 0;],'fill', [ 0;],'editID', [ 0;],'signalOrder', [ 1;])  canBus='CAN1'  queueSize=1  payloadMask=[]  payloadValue=[]  period=0  showID=0  label=0  idMask=hex2dec('1FFFFFFF')  fill=0  id=1515  showRaw=0  signalOrder=1  signalInfo={{struct('Name', 'CMU2_Tcell_T09','Startbit', [ 0;],'SignalSize', [ 8;],'ByteOrder', 'BigEndian','ValueType', 'UNSIGNED','Class', 'uint8','Signed', [ 0;],'Factor', [ 1;],'Offset', [ 0;],'Min', [ 0;],'Max', [ 0;],'Units', '','Comment', '','StartBit', [ 0;]),struct('Name', 'CMU2_Tcell_T10','Startbit', [ 0;],'SignalSize', [ 8;],'ByteOrder', 'BigEndian','ValueType', 'UNSIGNED','Class', 'uint8','Signed', [ 0;],'Factor', [ 1;],'Offset', [ 0;],'Min', [ 0;],'Max', [ 0;],'Units', '','Comment', '','StartBit', [ 8;]),struct('Name', 'CMU2_Tcell_T11','Startbit', [ 0;],'SignalSize', [ 8;],'ByteOrder', 'BigEndian','ValueType', 'UNSIGNED','Class', 'uint8','Signed', [ 0;],'Factor', [ 1;],'Offset', [ 0;],'Min', [ 0;],'Max', [ 0;],'Units', '','Comment', '','StartBit', [ 16;]),struct('Name', 'CMU2_Tcell_T12','Startbit', [ 0;],'SignalSize', [ 8;],'ByteOrder', 'BigEndian','ValueType', 'UNSIGNED','Class', 'uint8','Signed', [ 0;],'Factor', [ 1;],'Offset', [ 0;],'Min', [ 0;],'Max', [ 0;],'Units', '','Comment', '','StartBit', [ 24;]),struct('Name', 'CMU2_Tcell_T13','Startbit', [ 0;],'SignalSize', [ 8;],'ByteOrder', 'BigEndian','ValueType', 'UNSIGNED','Class', 'uint8','Signed', [ 0;],'Factor', [ 1;],'Offset', [ 0;],'Min', [ 0;],'Max', [ 0;],'Units', '','Comment', '','StartBit', [ 32;]),struct('Name', 'CMU2_Tcell_T14','Startbit', [ 0;],'SignalSize', [ 8;],'ByteOrder', 'BigEndian','ValueType', 'UNSIGNED','Class', 'uint8','Signed', [ 0;],'Factor', [ 1;],'Offset', [ 0;],'Min', [ 0;],'Max', [ 0;],'Units', '','Comment', '','StartBit', [ 40;]),struct('Name', 'CMU2_Tcell_T15','Startbit', [ 0;],'SignalSize', [ 8;],'ByteOrder', 'BigEndian','ValueType', 'UNSIGNED','Class', 'uint8','Signed', [ 0;],'Factor', [ 1;],'Offset', [ 0;],'Min', [ 0;],'Max', [ 0;],'Units', '','Comment', '','StartBit', [ 48;]),struct('Name', 'CMU2_Tcell_T16','Startbit', [ 0;],'SignalSize', [ 8;],'ByteOrder', 'BigEndian','ValueType', 'UNSIGNED','Class', 'uint8','Signed', [ 0;],'Factor', [ 1;],'Offset', [ 0;],'Min', [ 0;],'Max', [ 0;],'Units', '','Comment', '','StartBit', [ 56;])}}
      settings: SourceProductName=Raptor
  raptor_data_read : Raptor_lib/Data Storage/raptor_data_read  dataName='Rx_0x200C6A2_Cell_9_Temp'  dataShape=Scalar  idxSource=Input  idxRow=1  idxCol=1
      settings: SourceProductName=Raptor
  raptor_data_read1 : Raptor_lib/Data Storage/raptor_data_read  dataName='Rx_0x200C6A2_Cell_10_Temp'  dataShape=Scalar  idxSource=Input  idxRow=1  idxCol=1
      settings: SourceProductName=Raptor
  raptor_data_read2 : Raptor_lib/Data Storage/raptor_data_read  dataName='Rx_0x200C6A2_Cell_11_Temp'  dataShape=Scalar  idxSource=Input  idxRow=1  idxCol=1
      settings: SourceProductName=Raptor
  raptor_data_read3 : Raptor_lib/Data Storage/raptor_data_read  dataName='Rx_0x200C6A2_Cell_12_Temp'  dataShape=Scalar  idxSource=Input  idxRow=1  idxCol=1
      settings: SourceProductName=Raptor
  raptor_data_read4 : Raptor_lib/Data Storage/raptor_data_read  dataName='Rx_0x200C7A2_Cell_13_Temp'  dataShape=Scalar  idxSource=Input  idxRow=1  idxCol=1
      settings: SourceProductName=Raptor
  raptor_data_read5 : Raptor_lib/Data Storage/raptor_data_read  dataName='Rx_0x200C7A2_Cell_14_Temp'  dataShape=Scalar  idxSource=Input  idxRow=1  idxCol=1
      settings: SourceProductName=Raptor
  raptor_data_read6 : Raptor_lib/Data Storage/raptor_data_read  dataName='Rx_0x200C7A2_Cell_15_Temp'  dataShape=Scalar  idxSource=Input  idxRow=1  idxCol=1
      settings: SourceProductName=Raptor
  raptor_data_read7 : Raptor_lib/Data Storage/raptor_data_read  dataName='Rx_0x200C7A2_Cell_16_Temp'  dataShape=Scalar  idxSource=Input  idxRow=1  idxCol=1
      settings: SourceProductName=Raptor
  wires:
  raptor_data_read7/1 -> Fcn8/1
  Data Type Conversion5/1 -> raptor_can_txmsg/5
  Fcn4/1 -> Data Type Conversion4/1
  Fcn1/1 -> Data Type Conversion1/1
  Fcn8/1 -> Data Type Conversion8/1
  Data Type Conversion1/1 -> raptor_can_txmsg/2
  Data Type Conversion4/1 -> raptor_can_txmsg/4
  Data Type Conversion7/1 -> raptor_can_txmsg/7
  Fcn3/1 -> Data Type Conversion2/1
  Fcn6/1 -> Data Type Conversion6/1
  Fcn7/1 -> Data Type Conversion7/1
  raptor_data_read1/1 -> Fcn1/1
  Data Type Conversion6/1 -> raptor_can_txmsg/6
  raptor_data_read6/1 -> Fcn7/1
  Fcn2/1 -> Data Type Conversion3/1
  Data Type Conversion2/1 -> raptor_can_txmsg/3
  Data Type Conversion3/1 -> raptor_can_txmsg/1
  Fcn5/1 -> Data Type Conversion5/1
  Data Type Conversion8/1 -> raptor_can_txmsg/8
  raptor_data_read4/1 -> Fcn5/1
  raptor_data_read2/1 -> Fcn3/1
  raptor_data_read5/1 -> Fcn6/1
  raptor_data_read/1 -> Fcn2/1
  raptor_data_read3/1 -> Fcn4/1

== system EPT/Foreground_TimeBase_5ms/CAN/CAN1_exec/BCU vs RMDA-BMS/RollingCount ==
  In1 : Inport
  Add : Sum
  Constant1 : Constant
  Constant3 : Constant
  Data Type Conversion : DataTypeConversion
  NOT : Logic  Operator=NOT  IconShape=distinctive  AllPortsSameDT=off  OutDataTypeStr=boolean
  Relational Operator : RelationalOperator  Operator=>  OutDataTypeStr=boolean  RndMeth=Simplest
  Switch : Switch  Criteria=u2 > Threshold
  Unit Delay : UnitDelay  SampleTime=-1  HasFrameUpgradeWarning=on
  Out1 : Outport  VectorParamsAs1DForOutWhenUnconnected=off
  wires:
  Constant1/1 -> Switch/3
  In1/1 -> Relational Operator/2
  Switch/1 -> Unit Delay/1, Data Type Conversion/1
  NOT/1 -> Switch/2
  Add/1 -> Relational Operator/1, Switch/1
  Relational Operator/1 -> NOT/1
  Constant3/1 -> Add/2
  Unit Delay/1 -> Add/1
  Data Type Conversion/1 -> Out1/1

== system EPT/Foreground_TimeBase_5ms/CAN/CAN1_exec/BCU-CMU/CMU_Task ==
  Constant7 : Constant  Value=15
  Logical Operator{1..4} (4 alike) : Logic  AllPortsSameDT=off  OutDataTypeStr=boolean
  NOT : Logic  Operator=NOT  IconShape=distinctive  AllPortsSameDT=off  OutDataTypeStr=boolean
  Relational Operator{,1..3} (4 alike) : RelationalOperator  Operator===  OutDataTypeStr=boolean  RndMeth=Simplest
  Rem : Math  Operator=rem  SaturateOnIntegerOverflow=on
  Rem1 : Math  Operator=rem  SaturateOnIntegerOverflow=on
  Rem2 : Math  Operator=rem  SaturateOnIntegerOverflow=on
  RollingCount : Subsystem
  RollingCount1 : Subsystem
  Rx B0-B1 : Subsystem  TreatAsAtomicUnit=on
  Rx B2&(Ba-Bb) : Subsystem  TreatAsAtomicUnit=on
  Rx C0-C3 : Subsystem  TreatAsAtomicUnit=on
  Rx C4-C7 : Subsystem  TreatAsAtomicUnit=on
  Tx B0-B1 : Subsystem  TreatAsAtomicUnit=on
  Tx B2&(BA-BB) : Subsystem  TreatAsAtomicUnit=on
  Tx C0-C3 : Subsystem  TreatAsAtomicUnit=on
  Tx C4-C7 : Subsystem  TreatAsAtomicUnit=on
  Variable Integer Delay{,1..3} (4 alike) : Delay  DelayLengthSource=Input port
      settings: InputPortMap=u0,p1
  raptor_adjustment : Raptor_lib/Data Storage/raptor_adjustment  paramName='Cal_CMU_Raw_Data_Viewer'  nameSource=Parameter  initValue=1  dataType=boolean  storage=Calibration  calDispType=Number  calEnum={'False', 'True'}  calGain=1.0  calOffset=0.0  calMax=inf  calMin=-inf  calFormat='-1'  calUnit=''  calHelp=''  calAccess=1  calFunction=raptor_xcp_function(gcb)  calDispHeaders=off  calColHeaders={'Col1' 'Col2' 'Col3'}  calRowHeaders={'Row1' 'Row2' 'Row3'}
      settings: SourceProductName=Raptor
  raptor_adjustment1 : Raptor_lib/Data Storage/raptor_adjustment  paramName='Cal_CMU_TDM3'  nameSource=Parameter  initValue=200  dataType=uint8  storage=Calibration  calDispType=Number  calEnum={'False', 'True'}  calGain=1.0  calOffset=0.0  calMax=inf  calMin=-inf  calFormat='-1'  calUnit=''  calHelp=''  calAccess=1  calFunction=raptor_xcp_function(gcb)  calDispHeaders=off  calColHeaders={'Col1' 'Col2' 'Col3'}  calRowHeaders={'Row1' 'Row2' 'Row3'}
      settings: SourceProductName=Raptor
  raptor_adjustment10 : Raptor_lib/Data Storage/raptor_adjustment  paramName='Cal_CMU_Broadcast'  nameSource=Parameter  initValue=0  dataType=boolean  storage=Calibration  calDispType=Number  calEnum={'False', 'True'}  calGain=1.0  calOffset=0.0  calMax=inf  calMin=-inf  calFormat='-1'  calUnit=''  calHelp=''  calAccess=1  calFunction=raptor_xcp_function(gcb)  calDispHeaders=off  calColHeaders={'Col1' 'Col2' 'Col3'}  calRowHeaders={'Row1' 'Row2' 'Row3'}
      settings: SourceProductName=Raptor
  raptor_adjustment2 : Raptor_lib/Data Storage/raptor_adjustment  paramName='Cal_CMU_TDM1'  nameSource=Parameter  initValue=10  dataType=uint8  storage=Calibration  calDispType=Number  calEnum={'False', 'True'}  calGain=1.0  calOffset=0.0  calMax=inf  calMin=-inf  calFormat='-1'  calUnit=''  calHelp=''  calAccess=1  calFunction=raptor_xcp_function(gcb)  calDispHeaders=off  calColHeaders={'Col1' 'Col2' 'Col3'}  calRowHeaders={'Row1' 'Row2' 'Row3'}
      settings: SourceProductName=Raptor
  raptor_adjustment3 : Raptor_lib/Data Storage/raptor_adjustment  paramName='Cal_CMU_TDM_BASE'  nameSource=Parameter  initValue=200  dataType=uint8  storage=Calibration  calDispType=Number  calEnum={'False', 'True'}  calGain=1.0  calOffset=0.0  calMax=inf  calMin=-inf  calFormat='-1'  calUnit=''  calHelp=''  calAccess=1  calFunction=raptor_xcp_function(gcb)  calDispHeaders=off  calColHeaders={'Col1' 'Col2' 'Col3'}  calRowHeaders={'Row1' 'Row2' 'Row3'}
      settings: SourceProductName=Raptor
  raptor_adjustment4 : Raptor_lib/Data Storage/raptor_adjustment  paramName='Cal_CMU_TDM1_REM'  nameSource=Parameter  initValue=7  dataType=uint8  storage=Calibration  calDispType=Number  calEnum={'False', 'True'}  calGain=1.0  calOffset=0.0  calMax=inf  calMin=-inf  calFormat='-1'  calUnit=''  calHelp=''  calAccess=1  calFunction=raptor_xcp_function(gcb)  calDispHeaders=off  calColHeaders={'Col1' 'Col2' 'Col3'}  calRowHeaders={'Row1' 'Row2' 'Row3'}
      settings: SourceProductName=Raptor
  raptor_adjustment5 : Raptor_lib/Data Storage/raptor_adjustment  paramName='Cal_CMU_TDM2'  nameSource=Parameter  initValue=100  dataType=uint8  storage=Calibration  calDispType=Number  calEnum={'False', 'True'}  calGain=1.0  calOffset=0.0  calMax=inf  calMin=-inf  calFormat='-1'  calUnit=''  calHelp=''  calAccess=1  calFunction=raptor_xcp_function(gcb)  calDispHeaders=off  calColHeaders={'Col1' 'Col2' 'Col3'}  calRowHeaders={'Row1' 'Row2' 'Row3'}
      settings: SourceProductName=Raptor
  raptor_adjustment6 : Raptor_lib/Data Storage/raptor_adjustment  paramName='Cal_CMU_TDM2_REM'  nameSource=Parameter  initValue=72  dataType=uint8  storage=Calibration  calDispType=Number  calEnum={'False', 'True'}  calGain=1.0  calOffset=0.0  calMax=inf  calMin=-inf  calFormat='-1'  calUnit=''  calHelp=''  calAccess=1  calFunction=raptor_xcp_function(gcb)  calDispHeaders=off  calColHeaders={'Col1' 'Col2' 'Col3'}  calRowHeaders={'Row1' 'Row2' 'Row3'}
      settings: SourceProductName=Raptor
  raptor_adjustment7 : Raptor_lib/Data Storage/raptor_adjustment  paramName='Cal_CMU_TDM3_REM1'  nameSource=Parameter  initValue=132  dataType=uint8  storage=Calibration  calDispType=Number  calEnum={'False', 'True'}  calGain=1.0  calOffset=0.0  calMax=inf  calMin=-inf  calFormat='-1'  calUnit=''  calHelp=''  calAccess=1  calFunction=raptor_xcp_function(gcb)  calDispHeaders=off  calColHeaders={'Col1' 'Col2' 'Col3'}  calRowHeaders={'Row1' 'Row2' 'Row3'}
      settings: SourceProductName=Raptor
  raptor_adjustment8 : Raptor_lib/Data Storage/raptor_adjustment  paramName='Cal_CMU_TDM3_REM2'  nameSource=Parameter  initValue=162  dataType=uint8  storage=Calibration  calDispType=Number  calEnum={'False', 'True'}  calGain=1.0  calOffset=0.0  calMax=inf  calMin=-inf  calFormat='-1'  calUnit=''  calHelp=''  calAccess=1  calFunction=raptor_xcp_function(gcb)  calDispHeaders=off  calColHeaders={'Col1' 'Col2' 'Col3'}  calRowHeaders={'Row1' 'Row2' 'Row3'}
      settings: SourceProductName=Raptor
  raptor_adjustment9 : Raptor_lib/Data Storage/raptor_adjustment  paramName='Cal_CMU_Rx_DelayTime'  nameSource=Parameter  initValue=2  dataType=uint8  storage=Calibration  calDispType=Number  calEnum={'False', 'True'}  calGain=1.0  calOffset=0.0  calMax=inf  calMin=-inf  calFormat='-1'  calUnit=''  calHelp=''  calAccess=1  calFunction=raptor_xcp_function(gcb)  calDispHeaders=off  calColHeaders={'Col1' 'Col2' 'Col3'}  calRowHeaders={'Row1' 'Row2' 'Row3'}
      settings: SourceProductName=Raptor
  raptor_data_def1 : Raptor_lib/Data Storage/raptor_data_def  dataName='EPT_RDCMD_OFFSET'  initValue=0  dataType=uint8  storage=Volatile (RAM)  calVisible=on  calType=Adjustment  calDispType=Number  calEnum={'False', 'True'}  calGain=1.0  calOffset=0  calMin=-inf  calMax=inf  calFormat='-1'  calUnit=''  calHelp=''  calAccess=1  calFunction=raptor_xcp_function(gcb)  calDispHeaders=off  calColHeaders={'Col1' 'Col2' 'Col3'}  calRowHeaders={'Row1' 'Row2' 'Row3'}
      settings: SourceProductName=Raptor
  raptor_data_def11 : Raptor_lib/Data Storage/raptor_data_def  dataName='EPT_RDCMD_CMU_ID'  initValue=0  dataType=uint8  storage=Volatile (RAM)  calVisible=on  calType=Adjustment  calDispType=Number  calEnum={'False', 'True'}  calGain=1.0  calOffset=0  calMin=-inf  calMax=inf  calFormat='-1'  calUnit=''  calHelp=''  calAccess=1  calFunction=raptor_xcp_function(gcb)  calDispHeaders=off  calColHeaders={'Col1' 'Col2' 'Col3'}  calRowHeaders={'Row1' 'Row2' 'Row3'}
      settings: SourceProductName=Raptor
  raptor_data_def3 : Raptor_lib/Data Storage/raptor_data_def  dataName='EPT_RDCMD_HOST_ID'  initValue=0  dataType=uint8  storage=Volatile (RAM)  calVisible=on  calType=Adjustment  calDispType=Number  calEnum={'False', 'True'}  calGain=1.0  calOffset=0  calMin=-inf  calMax=inf  calFormat='-1'  calUnit=''  calHelp=''  calAccess=1  calFunction=raptor_xcp_function(gcb)  calDispHeaders=off  calColHeaders={'Col1' 'Col2' 'Col3'}  calRowHeaders={'Row1' 'Row2' 'Row3'}
      settings: SourceProductName=Raptor
  raptor_data_def4 : Raptor_lib/Data Storage/raptor_data_def  dataName='EPT_RDCMD_RC'  initValue=0  dataType=uint8  storage=Volatile (RAM)  calVisible=on  calType=Adjustment  calDispType=Number  calEnum={'False', 'True'}  calGain=1.0  calOffset=0  calMin=-inf  calMax=inf  calFormat='-1'  calUnit=''  calHelp=''  calAccess=1  calFunction=raptor_xcp_function(gcb)  calDispHeaders=off  calColHeaders={'Col1' 'Col2' 'Col3'}  calRowHeaders={'Row1' 'Row2' 'Row3'}
      settings: SourceProductName=Raptor
  raptor_data_write20 : Raptor_lib/Data Storage/raptor_data_write  dataName='EPT_RDCMD_RC'  dataShape=Scalar  idxSource=Input Port  idxRow=1  idxCol=1
      settings: SourceProductName=Raptor
  wires:
  Rem/1 -> Relational Operator/1
  RollingCount1/1(Out1) -> raptor_data_write20/1
  raptor_adjustment3/1 -> RollingCount/1(In1)
  Relational Operator/1 -> Logical Operator3/1, Variable Integer Delay/1
  raptor_adjustment5/1 -> Rem1/2
  Relational Operator1/1 -> Logical Operator4/1, Variable Integer Delay1/1
  Variable Integer Delay/1 -> Rx B0-B1/Trigger
  Constant7/1 -> RollingCount1/1(In1)
  Variable Integer Delay1/1 -> Rx B2&(Ba-Bb)/Trigger
  raptor_adjustment2/1 -> Rem/2
  raptor_adjustment/1 -> Logical Operator2/1, Logical Operator1/2
  Rem1/1 -> Relational Operator1/1
  Relational Operator3/1 -> Logical Operator1/1
  Logical Operator1/1 -> Variable Integer Delay3/1, Tx C4-C7/Trigger
  Relational Operator2/1 -> Logical Operator2/2
  Logical Operator2/1 -> Variable Integer Delay2/1, Tx C0-C3/Trigger
  Variable Integer Delay3/1 -> Rx C4-C7/Trigger
  Variable Integer Delay2/1 -> Rx C0-C3/Trigger
  RollingCount/1(Out) -> Rem2/1, Rem1/1, Rem/1
  Rem2/1 -> Relational Operator3/1, Relational Operator2/1
  raptor_adjustment1/1 -> Rem2/2
  raptor_adjustment6/1 -> Relational Operator1/2
  raptor_adjustment4/1 -> Relational Operator/2
  raptor_adjustment7/1 -> Relational Operator2/2
  raptor_adjustment8/1 -> Relational Operator3/2
  raptor_adjustment9/1 -> Variable Integer Delay2/2, Variable Integer Delay1/2, Variable Integer Delay/2, Variable Integer Delay3/2
  raptor_adjustment10/1 -> NOT/1
  NOT/1 -> Logical Operator4/2, Logical Operator3/2
  Logical Operator3/1 -> Tx B0-B1/Trigger
  Logical Operator4/1 -> Tx B2&(BA-BB)/Trigger

== system EPT/Foreground_TimeBase_5ms/CAN/CAN1_exec/CountTrigger1/CycleTrigger ==
  In1 : Inport
  In2 : Inport  Port=2
  Add : Sum
  Add1 : Sum
  Add2 : Sum  Inputs=+-
  Constant1 : Constant
  Constant2 : Constant  Value=0
  Constant3 : Constant
  Data Type Conversion1 : DataTypeConversion
  Data Type Conversion2 : DataTypeConversion
  Display : Display
  Relational Operator1 : RelationalOperator  OutDataTypeStr=boolean  RndMeth=Simplest
  Scope : Scope
  Scope1 : Scope
  Scope2 : Scope
  Switch : Switch  Threshold=1
  Unit Delay : UnitDelay  SampleTime=-1  HasFrameUpgradeWarning=on
  Unit Delay1 : UnitDelay  SampleTime=-1  HasFrameUpgradeWarning=on
  Trigger : Outport  VectorParamsAs1DForOutWhenUnconnected=off
  wires:
  Add/1 -> Switch/1
  In1/1 -> Data Type Conversion2/1
  Unit Delay/1 -> Add/1
  Switch/1 -> Relational Operator1/1, Scope1/1, Unit Delay/1
  Add1/1 -> Scope/1, Unit Delay1/1, Display/1
  Unit Delay1/1 -> Add1/1
  Constant1/1 -> Add1/2
  Relational Operator1/1 -> Scope2/1, Trigger/1
  Data Type Conversion1/1 -> Relational Operator1/2
  Constant2/1 -> Switch/3
  Data Type Conversion2/1 -> Add/2, Switch/2
  Add2/1 -> Data Type Conversion1/1
  In2/1 -> Add2/1
  Constant3/1 -> Add2/2

== system EPT/Foreground_TimeBase_5ms/CAN/CAN1_exec/IVT/CountTrigger ==
  Counter : Inport
  Constant1 : Constant  Value=0
  Constant3 : Constant
  CycleTrigger : Subsystem
  Switch : Switch  Threshold=1
  Unit Delay1 : UnitDelay  SampleTime=-1  HasFrameUpgradeWarning=on
  Unit Delay2 : UnitDelay  SampleTime=-1  HasFrameUpgradeWarning=on
  Tirgger : Outport  VectorParamsAs1DForOutWhenUnconnected=off
  wires:
  Unit Delay2/1 -> Tirgger/1
  Unit Delay1/1 -> CycleTrigger/1(In1)
  CycleTrigger/1(Trigger) -> Unit Delay2/1, Switch/2
  Counter/1 -> CycleTrigger/2(In2)
  Constant1/1 -> Switch/1
  Constant3/1 -> Switch/3
  Switch/1 -> Unit Delay1/1

== system EPT/Foreground_TimeBase_5ms/CAN/CAN1_exec/IVT/CountTrigger1 ==
  Counter : Inport
  Constant1 : Constant  Value=0
  Constant3 : Constant
  CycleTrigger : Subsystem
  Switch : Switch  Threshold=1
  Unit Delay1 : UnitDelay  SampleTime=-1  HasFrameUpgradeWarning=on
  Unit Delay2 : UnitDelay  SampleTime=-1  HasFrameUpgradeWarning=on
  Tirgger : Outport  VectorParamsAs1DForOutWhenUnconnected=off
  wires:
  Switch/1 -> Unit Delay1/1
  Constant3/1 -> Switch/3
  Constant1/1 -> Switch/1
  Counter/1 -> CycleTrigger/2(In2)
  CycleTrigger/1(Trigger) -> Switch/2, Unit Delay2/1
  Unit Delay1/1 -> CycleTrigger/1(In1)
  Unit Delay2/1 -> Tirgger/1
